simulink model "IoTKeren_PemodelanSistemSimulink"  (R2021a)
settings: Solver=VariableStepAuto  StartTime=0.0  StopTime=121  RelTol=1e-3
undefined symbols (not defined in the file or in its folder): sigbuilder_block
settings Model: Creator=Hype G12  LastModifiedBy=Hype G12

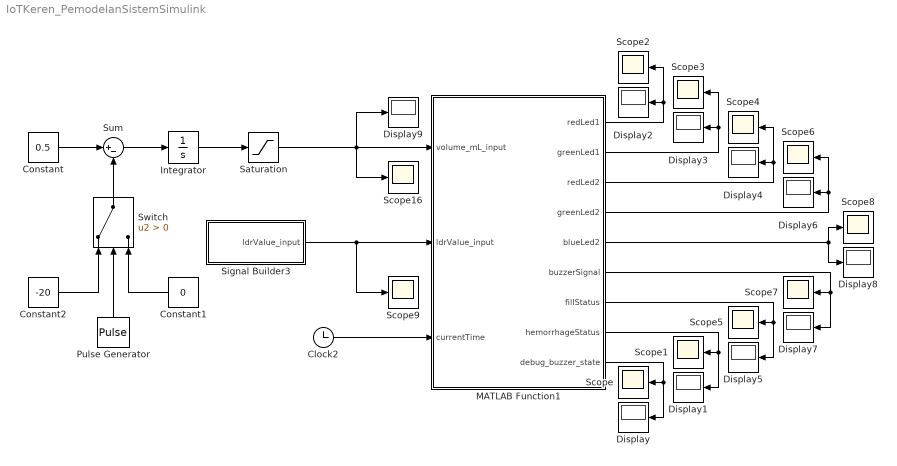
== system IoTKeren_PemodelanSistemSimulink ==
  Clock2 : Clock
  Constant : Constant  Value=0.5
  Constant1 : Constant  Value=0
  Constant2 : Constant  Value=-20
  Display{,1..9} (10 alike) : Display
  Integrator : Integrator
  MATLAB Function1 : MATLAB Function  TreatAsAtomicUnit=on  SystemSampleTime=0.01
  Pulse Generator : DiscretePulseGenerator  PulseType=Time based  Period=100  PhaseDelay=50
  Saturation : Saturate  UpperLimit=100.0  LowerLimit=0.0
  Scope{,1..9,16} (11 alike) : Scope
  Signal Builder3 : Subsystem  Tag=STV Subsys  LoadFcn=sigbuilder_block('load');  StartFcn=sigbuilder_block('start');  StopFcn=sigbuilder_block('stop');  ClipboardFcn=sigbuilder_block('clipboard');  mask(Sigbuilder block){tuvar=[0:10]}
      mask help: Simulink:masks:SigbuilderBlock_MD
      mask init:
      | if ~strcmp(get_param(bdroot(gcbh),'SimulationStatus'),'stopped') tuvar = sigbuilder_block('maskInit'); end
      settings: CopyFcn=sigbuilder_block('copy');  DeleteFcn=sigbuilder_block('delete');  ModelCloseFcn=sigbuilder_block('modelClose');  PreSaveFcn=sigbuilder_block('preSave');  PauseFcn=sigbuilder_block('pause');  ContinueFcn=sigbuilder_block('continue');  NameChangeFcn=sigbuilder_block('namechange');  OpenFcn=sigbuilder_block('open',[187 18 550.5 362.5 ]);  CloseFcn=sigbuilder_block('close');
      mask Display: plot(0, 0, 100, 100,[2, 2, 32, 32, 2], [68, 8, 8, 68, 68],[32, 2], [38, 38], [32, 19, 2],[53, 60, 44], [32, 17, 17, 2],[16, 16, 31, 31]);txt = getActiveGroup(gcbh);text(2, 100, txt,'verticalAlignment', 'top');
  Sum : Sum  Inputs=|+-
  Switch : Switch  Criteria=u2 > Threshold
  wires:
  Signal Builder3/1(ldrValue_input) -> Scope9/1, MATLAB Function1/2(ldrValue_input)
  Clock2/1 -> MATLAB Function1/3(currentTime)
  Constant/1 -> Sum/1
  Switch/1 -> Sum/2
  Sum/1 -> Integrator/1
  Integrator/1 -> Saturation/1
  Constant2/1 -> Switch/1
  Constant1/1 -> Switch/3
  Saturation/1 -> Display9/1, Scope16/1, MATLAB Function1/1(volume_mL_input)
  Pulse Generator/1 -> Switch/2
  MATLAB Function1/9(debug_buzzer_state) -> Display/1, Scope/1
  MATLAB Function1/8(hemorrhageStatus) -> Display1/1, Scope1/1
  MATLAB Function1/1(redLed1) -> Scope2/1, Display2/1
  MATLAB Function1/2(greenLed1) -> Scope3/1, Display3/1
  MATLAB Function1/3(redLed2) -> Scope4/1, Display4/1
  MATLAB Function1/7(fillStatus) -> Display5/1, Scope5/1
  MATLAB Function1/6(buzzerSignal) -> Display7/1, Scope7/1
  MATLAB Function1/4(greenLed2) -> Scope6/1, Display6/1
  MATLAB Function1/5(blueLed2) -> Display8/1, Scope8/1

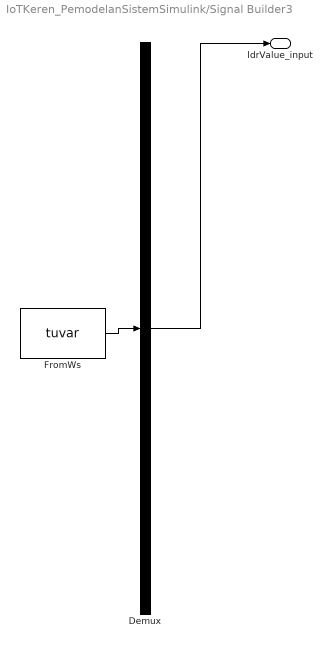
== system IoTKeren_PemodelanSistemSimulink/Signal Builder3 ==
  Demux : Demux  Tag=STV Demux  Outputs=1
      settings: DisplayOption=none
  FromWs : FromWorkspace  Tag=STV FromWs  VariableName=tuvar
      SigBuilderData=|
      | common.afterFinalStr = 'Extrapolate'
      | common.sampleTime = 0
      | dataSet(1).timeRange = [0 150]
      | dataSet(1).name = 'Tidak Terdeksi Darah'
      | dataSet(2).timeRange = [0 150]
      | dataSet(2).name = 'Terdeteksi Darah'
      | sbobj.Groups(1).Name = 'Tidak Terdeksi Darah'
      | sbobj.Groups(1).Signals.Name = 'ldrValue_input'
      | sbobj.Groups(1).Signals.XData = [0 150]
      | sbobj.Groups(1).Signals.YData = [1500 1500]
      | sbobj.Groups(1).TimeRange = [0 150]
      | sbobj.Groups(2).Name = 'Terdeteksi Darah'
      | sbobj.Groups(2).Signals.Name = 'ldrValue_input'
      | sbobj.Groups(2).Signals.XData = [0 150]
      | sbobj.Groups(2).Signals.YData = [500 500]
      | sbobj.Groups(2).TimeRange = [0 150]
  ldrValue_input : Outport  Tag=STV Outport
  wires:
  Demux/1 -> ldrValue_input/1
  FromWs/1 -> Demux/1

== matlab function IoTKeren_PemodelanSistemSimulink/MATLAB Function1 ==
  data: volume_mL_input input; redLed1 output; ldrValue_input input; greenLed1 output; redLed2 output; greenLed2 output; blueLed2 output; buzzerSignal output; fillStatus output; hemorrhageStatus output; currentTime input; debug_buzzer_state output
function [redLed1, greenLed1, redLed2, greenLed2, blueLed2, buzzerSignal, fillStatus, hemorrhageStatus, debug_buzzer_state] = urineMonitor(volume_mL_input, ldrValue_input, currentTime)

    % Variabel persisten untuk status buzzer dan timer/penghitung
    persistent buzzer_state;            % 0: Mati, 1: Berbunyi untuk penuh, 2: Berosilasi untuk pendarahan
    persistent buzzer_hemorrhage_timer; % Timer untuk osilasi 1 menit
    persistent buzzer_full_count;       % Penghitung untuk 3 bunyi bip
    persistent full_beep_timer;         % Timer untuk bip/jeda individual
    persistent full_beep_state;         % 0: idle, 1: berbunyi, 2: jeda untuk FSM 3-bip

    % Inisialisasi variabel persisten jika kosong (panggilan pertama fungsi)
    if isempty(buzzer_state)
        buzzer_state = 0;
    end
    if isempty(buzzer_hemorrhage_timer)
        buzzer_hemorrhage_timer = 0;
    end
    if isempty(buzzer_full_count)
        buzzer_full_count = 0;
    end
    if isempty(full_beep_timer)
        full_beep_timer = 0;
    end
    if isempty(full_beep_state)
        full_beep_state = 0;
    end

    % Definisikan konstanta
    LDR_THRESHOLD = 1000; % Ambang batas untuk LDR (lebih tinggi berarti lebih sedikit darah)
    LEVEL_KOSONG = 0;
    LEVEL_HAMPIR_PENUH_START = 70.0; % Disesuaikan dari LEVEL_AMAN_MAX
    LEVEL_PENUH_START = 90.0; % Sesuai dengan LEVEL_HAMPIR_PENUH Anda
    MAX_VOLUME = 100.0; % Asumsi volume maks untuk status "Penuh"

    % Inisialisasi output untuk langkah simulasi saat ini (selalu pastikan nilai default)
    redLed1 = 0;    % Untuk LED RGB (Pendarahan)
    greenLed1 = 0;  % Untuk LED RGB (Pendarahan)
    redLed2 = 0;    % Untuk LED Bar Graph (Level Pengisian - Merah)
    greenLed2 = 0;  % Untuk LED Bar Graph (Level Pengisian - Hijau)
    blueLed2 = 0;   % Untuk LED Bar Graph (Level Pengisian - Biru) - OUTPUT BARU
    buzzerSignal = 0;
    fillStatus = 0;     % 0: AMAN (Kosong...Hampir Penuh), 1: Hampir Penuh, 2: PENUH
    hemorrhageStatus = 0; % 0: Tidak Tercampur Darah, 1: Tercampur Darah

    % --- 1. PROSES LOGIKA SENSOR ---

    % Deteksi Hematuria (LDR & LED RGB)
    % isUrineNormal bernilai true jika nilai LDR tinggi (tidak ada darah), false jika rendah (darah terdeteksi)
    isUrineNormal = (ldrValue_input > LDR_THRESHOLD);
    if ~isUrineNormal % Tercampur darah (LDR rendah)
        redLed1 = 1;    % LED RGB Merah
        greenLed1 = 0;
        hemorrhageStatus = 1; % Status: Tercampur Darah
    else % Tidak tercampur darah (LDR tinggi)
        redLed1 = 0;
        greenLed1 = 1;  % LED RGB Hijau
        hemorrhageStatus = 0; % Status: Tidak Tercampur Darah
    end

    % Deteksi Level Urin (Load Cell & LED Bar Graph)
    if volume_mL_input >= LEVEL_PENUH_START && volume_mL_input <= MAX_VOLUME
        fillStatus = 2; % Status: PENUH
        redLed2 = 1;    % LED Bar Graph Merah
        greenLed2 = 0;
        blueLed2 = 0;
    elseif volume_mL_input >= LEVEL_HAMPIR_PENUH_START && volume_mL_input < LEVEL_PENUH_START
        fillStatus = 1; % Status: Hampir Penuh
        redLed2 = 0;
        greenLed2 = 0;
        blueLed2 = 1;   % LED Bar Graph Biru
    else % volume_mL_input < LEVEL_HAMPIR_PENUH_START (Kosong...Hampir Penuh)
        fillStatus = 0; % Status: AMAN
        redLed2 = 0;
        greenLed2 = 1;  % LED Bar Graph Hijau
        blueLed2 = 0;
    end

    % --- 2. KONTROL AKTUATOR (BUZZER) ---

    % TAHAP 1: Tentukan mode buzzer yang diinginkan berdasarkan prioritas
    % current_buzzer_mode: 0=Mati, 1=Bip Penuh, 2=Osilasi Pendarahan, 3=Bip Hampir Penuh (Baru)
    current_buzzer_mode = 0; % Default: Mati

    if hemorrhageStatus == 1 % Pendarahan memiliki prioritas tertinggi
        current_buzzer_mode = 2;
    elseif fillStatus == 2 % Penuh (prioritas kedua setelah pendarahan)
        current_buzzer_mode = 1;
    elseif fillStatus == 1 % Hampir Penuh (prioritas ketiga)
        current_buzzer_mode = 3; % Mode baru untuk buzzer "Hampir Penuh"
    end

    % TAHAP 2: Kelola status buzzer dan sinyal output berdasarkan current_buzzer_mode
    if current_buzzer_mode == 2 % Buzzer dalam mode Pendarahan (Osilasi)
        % Jika baru masuk mode ini atau kembali dari mode lain
        if buzzer_state ~= 2
            buzzer_state = 2; % Atur status
            buzzer_hemorrhage_timer = currentTime; % Mulai timer osilasi
            % Reset logika bip penuh jika pendarahan mengambil alih
            buzzer_full_count = 0;
            full_beep_state = 0;
            full_beep_timer = 0; % Pastikan timer penuh juga direset
        end
        
        % Lakukan osilasi selama 1 menit (60 detik)
        if (currentTime - buzzer_hemorrhage_timer) < 60
            % Osilasi kotak sederhana (misal ON 0.1s, OFF 0.1s, frekuensi 5Hz)
            % Ini menciptakan suara ON/OFF yang cepat selama 1 menit
            if mod(floor(currentTime * 5), 2) == 0 
                buzzerSignal = 1; % Buzzer ON
            else
                buzzerSignal = 0; % Buzzer OFF
            end
        else % 1 menit telah berlalu, hentikan osilasi
            buzzer_state = 0; % Matikan status buzzer
            buzzerSignal = 0;
            buzzer_hemorrhage_timer = 0; % Reset timer
        end

    elseif current_buzzer_mode == 1 % Buzzer dalam mode Penuh (3 Bip)
        % Jika baru masuk mode ini atau urutan bip perlu dimulai/dilanjutkan
        if buzzer_state ~= 1
            buzzer_state = 1; % Atur status
            % Reset timer pendarahan jika mode penuh mengambil alih
            buzzer_hemorrhage_timer = 0; % Penting untuk memastikan bersih dari mode sebelumnya
            % Pastikan urutan 3-bip dimulai dari awal
            buzzer_full_count = 0;
            full_beep_state = 0;
            full_beep_timer = 0;
        end
        
        % Kelola urutan 3-bip menggunakan Finite State Machine (FSM)
        switch full_beep_state
            case 0 % Idle, siap memulai/melanjutkan 3 bip
                if buzzer_full_count < 3 % Jika masih ada bip yang harus dilakukan
                    full_beep_state = 1; % Pindah ke status berbunyi
                    full_beep_timer = currentTime; % Mulai timer untuk durasi bip
                    buzzerSignal = 1; % Buzzer ON (memulai bip)
                    buzzer_full_count = buzzer_full_count + 1; % Tambah penghitung bip
                else
                    buzzerSignal = 0; % 3 bip selesai
                    buzzer_state = 0; % Kembali ke idle (matikan mode buzzer)
                    buzzer_full_count = 0; % Reset penghitung bip untuk event berikutnya
                    full_beep_state = 0; % Reset FSM untuk event berikutnya
                    full_beep_timer = 0; % Reset timer
                end
            case 1 % Status Berbunyi (buzzer ON)
                if (currentTime - full_beep_timer) < 0.2 % Durasi bip (0.2 detik)
                    buzzerSignal = 1;
                else
                    full_beep_state = 2; % Pindah ke status jeda
                    full_beep_timer = currentTime; % Mulai timer untuk durasi jeda
                    buzzerSignal = 0; % Buzzer OFF
                end
            case 2 % Status Jeda antar bip (buzzer OFF)
                if (currentTime - full_beep_timer) < 0.3 % Durasi jeda (0.3 detik)
                    buzzerSignal = 0;
                else
                    full_beep_state = 0; % Kembali ke status idle untuk memeriksa bip berikutnya
                end
        end

    elseif current_buzzer_mode == 3 % Buzzer dalam mode Hampir Penuh (Satu Bip) - LOGIKA BARU
        % Logika ini memastikan satu bip pendek saat transisi ke "Hampir Penuh"
        % dan kemudian tetap mati kecuali status berubah atau kembali ke "Hampir Penuh".
        if buzzer_state ~= 3
            buzzer_state = 3; % Atur status untuk "Hampir Penuh"
            buzzer_full_count = 0; % Reset penghitung bip penuh
            full_beep_state = 0; % Reset FSM bip penuh
            buzzer_hemorrhage_timer = 0; % Reset timer pendarahan
            
            % Picu satu bip pendek
            buzzerSignal = 1; % Buzzer ON
            full_beep_timer = currentTime; % Gunakan full_beep_timer untuk durasi bip pendek ini
        end

        % Matikan buzzer setelah durasi singkat untuk bip tunggal "Hampir Penuh"
        if buzzerSignal == 1 && (currentTime - full_beep_timer) >= 0.2 % Durasi bip 0.2 detik
            buzzerSignal = 0;
            % Setelah bip tunggal selesai, jaga buzzer_state sebagai 3 tetapi buzzerSignal sebagai 0
            % Ini mencegah bip terus menerus untuk "Hampir Penuh"
        end

    else % current_buzzer_mode == 0 (Tidak ada kondisi buzzer aktif)
        buzzer_state = 0; % Pastikan buzzer OFF
        buzzerSignal = 0;
        buzzer_hemorrhage_timer = 0; % Reset semua timer/penghitung
        buzzer_full_count = 0;
        full_beep_state = 0;
        full_beep_timer = 0;
    end
    % AKHIR logika buzzer

    % Output variabel debug
    debug_buzzer_state = buzzer_state;

end % AKHIR fungsi urineMonitor
